simulink model "Block_Diagram"  (R2022b)
settings: Solver=VariableStepAuto  StartTime=0.0  StopTime=10.0  RelTol=1e-3
values from neighbouring files (symbols this model uses):
  den = [1 0 -1]    [Workshop2_Hinf_control.m]
  den1 = [1 0.001]    [Workshop2_Hinf_control.m]
  den2 = [1 300]    [Workshop2_Hinf_control.m]
  num = 1    [Workshop2_Hinf_control.m]
  num1 = [1 1]    [Workshop2_Hinf_control.m]
  num2 = [1 3]    [Workshop2_Hinf_control.m]
settings Model: Creator=Akash  LastModifiedBy=Akash

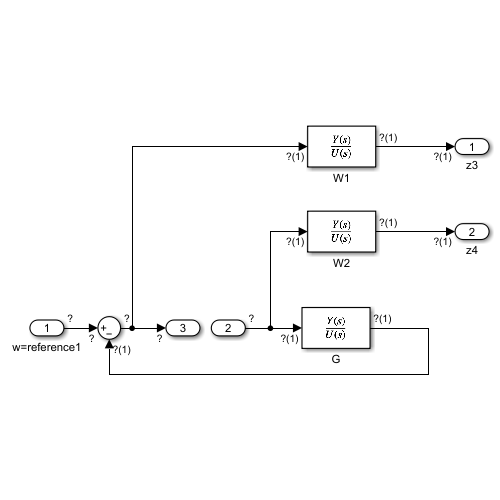
[thumbnail: Simulink's stored preview of the top-level diagram]
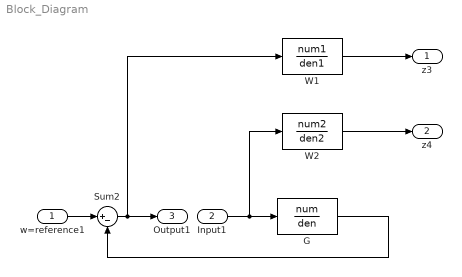
== system Block_Diagram ==
  w=reference1 : Inport
  Input1 : Inport  Port=2
  G : TransferFcn  Numerator=num  Denominator=den
  Sum2 : Sum  Inputs=|+-
  W1 : TransferFcn  Numerator=num1  Denominator=den1
  W2 : TransferFcn  Numerator=num2  Denominator=den2
  z3 : Outport
  z4 : Outport  Port=2
  Output1 : Outport  Port=3
  wires:
  Input1/1 -> G/1, W2/1
  W2/1 -> z4/1
  W1/1 -> z3/1
  Sum2/1 -> Output1/1, W1/1
  w=reference1/1 -> Sum2/1
  G/1 -> Sum2/2
